simulink model "bai6sml"  (R2015a)
settings: Solver=ode45  StartTime=0.0  StopTime=10.0  RelTol=1e-3
values from neighbouring files (symbols this model uses):
  b = [1;2;1]    [Bai1.m]    (also in Bai6.m = 2; bai2.m = [6; 9]; bai2b.m = [1; 2; 3; 4])
  c = [2;3;4]    [Bai1.m]    (also in Bai6.m = 100)
  m = 1    [Bai6.m]
libraries: simulink x1
settings Model: Creator=Tung  LastModifiedBy=Tung

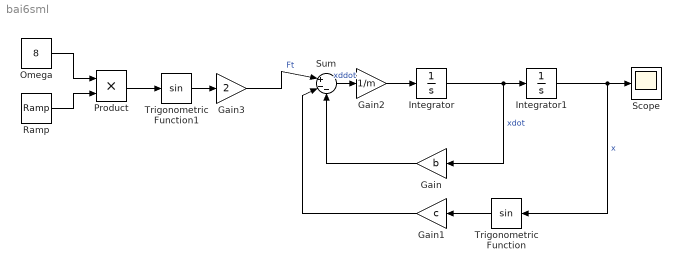
== system bai6sml ==
  Gain : Gain  Gain=b
  Gain1 : Gain  Gain=c
  Gain2 : Gain  Gain=1/m
  Gain3 : Gain  Gain=2
  Integrator : Integrator
  Integrator1 : Integrator
  Omega : Constant  Value=8
  Product : Product
  Ramp : simulink/Sources/Ramp  slope=1  start=0  X0=0
  Scope : Scope
  Sum : Sum  Inputs=|+--
  Trigonometric Function : Trigonometry
  Trigonometric Function1 : Trigonometry
  wires:
  Integrator/1 -> Gain/1, Integrator1/1  "xdot"
  Integrator1/1 -> Trigonometric Function/1, Scope/1  "x"
  Sum/1 -> Gain2/1  "xddot"
  Gain/1 -> Sum/3
  Trigonometric Function/1 -> Gain1/1
  Gain1/1 -> Sum/2
  Gain2/1 -> Integrator/1
  Omega/1 -> Product/1
  Ramp/1 -> Product/2
  Product/1 -> Trigonometric Function1/1
  Trigonometric Function1/1 -> Gain3/1
  Gain3/1 -> Sum/1  "Ft"
